simulink model "Power_Factor_Correction_using_CAPACITOR_BANK"  (R2022b)
settings: Solver=VariableStepAuto  StartTime=0.0  StopTime=0.2  RelTol=1e-3
undefined symbols (not defined in the file): D1, Delta
libraries: spsThreePhaseParallelRLCLoadLib x7, spsThreePhaseBreakerLib x6, spsPower3phInstantaneousLib x1, spsThreePhaseTransformerTwoWindingsLib x1, spsThreePhaseVIMeasurementLib x1, spsThreePhaseSourceLib x1, spspowerguiLib x1
settings Model: Creator=shubham  LastModifiedBy=shubham

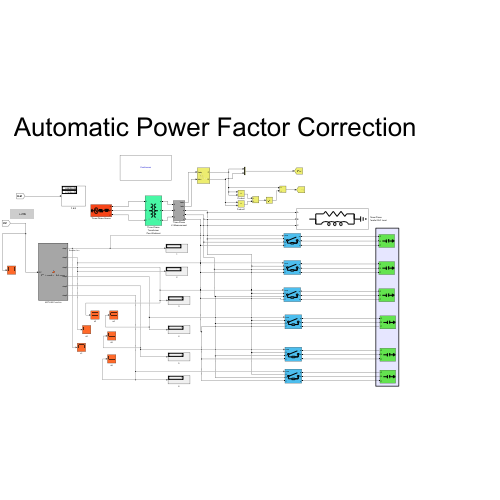
[thumbnail: Simulink's stored preview of the top-level diagram]
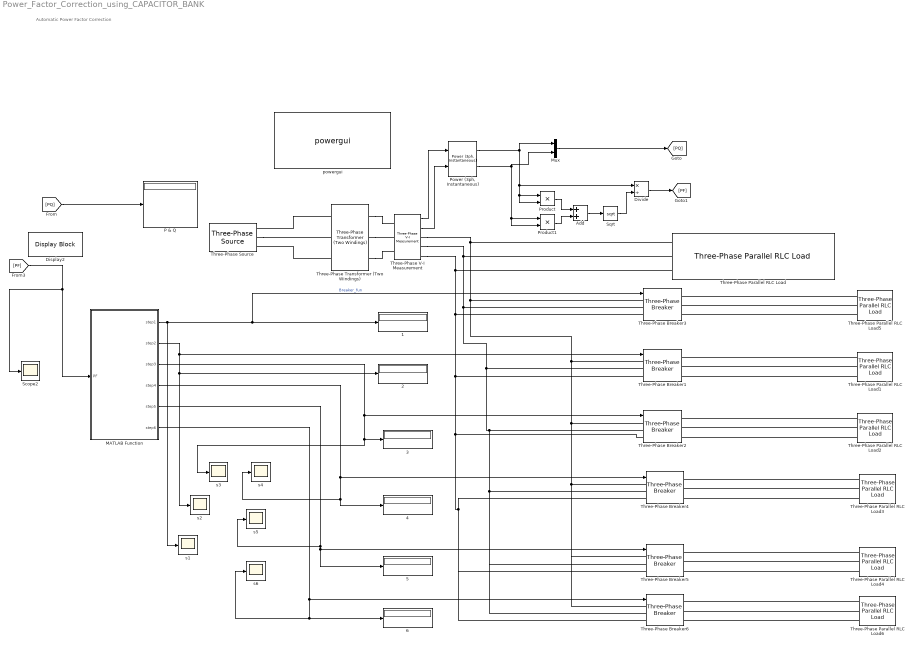
== system Power_Factor_Correction_using_CAPACITOR_BANK ==
  note: Automatic Power Factor Correction
  {1..6} (6 alike) : Display
      settings: Decimation=4
  Add : Sum
  Display2 : DisplayBlock  LabelPosition=Hide  Transparency=1  Layout=Fill available space
  Divide : Product  Inputs=*/
  MATLAB Function : MATLAB Function  TreatAsAtomicUnit=on
  Mux : Mux  Inputs=2
  P & Q : Display
      settings: Format=short_e  Decimation=4
  "Power (3ph, Instantaneous)" : spsPower3phInstantaneousLib/Power (3ph, Instantaneous)
  Product : Product
  Product1 : Product
  Scope2 : Scope
  Sqrt : Sqrt
  Three-Phase Parallel RLC Load : spsThreePhaseParallelRLCLoadLib/Three-Phase Parallel RLC Load  LConnTagsString=A|B|C  Configuration=Y (grounded)  NominalVoltage=6600  Vabc=[1e3 1e3 1e3]  Vabcp=[1e3 1e3 1e3]  NominalFrequency=50  UnbalancedPower=off  ActivePower=5000000  InductivePower=5845000  CapacitivePower=0  Pabc=[10e3 9e3 11e3]  QLabc=[100 90 110]  QCabc=[100 90 110]  Pabcp=[10e3 9e3 11e3]  QLabcp=[100 90 110]  QCabcp=[100 90 110]  Measurements=None  LoadType=constant Z
  Three-Phase Parallel RLC Load{1..6} (6 alike) : spsThreePhaseParallelRLCLoadLib/Three-Phase Parallel RLC Load  LConnTagsString=A|B|C  Configuration=Y (grounded)  NominalVoltage=6600  Vabc=[1e3 1e3 1e3]  Vabcp=[1e3 1e3 1e3]  NominalFrequency=50  UnbalancedPower=off  ActivePower=0  InductivePower=0  CapacitivePower=650000  Pabc=[10e3 9e3 11e3]  QLabc=[100 90 110]  QCabc=[100 90 110]  Pabcp=[10e3 9e3 11e3]  QLabcp=[100 90 110]  QCabcp=[100 90 110]  Measurements=None  LoadType=constant Z
  Three-Phase Transformer (Two Windings) : spsThreePhaseTransformerTwoWindingsLib/Three-Phase Transformer (Two Windings)  Winding1Connection=Delta (D1)  Winding2Connection=Yg  CoreType=Three single-phase transformers  SetSaturation=off  Hysteresis=off  DataFile='hysteresis'  SetInitialFlux=off  Measurements=None  UNITS=pu  NominalPower=[ 5e6 , 50 ]  Winding1=[ 33e3 , 0.002 , 0.08 ]  Winding2=[ 6.6e3 , 0.002 , 0.08 ]  Rm=500  Lm=500  L0=0.5  Saturation=[ 0,0 ; 0.0024,1.2 ; 1.0,1.52 ]  InitialFluxes=[ 0.8 , -0.8 , 0.7 ]  BreakLoop=off  DiscreteSolver=Trapezoidal iterative  DataType=off  TransfoNumber=1
  Three-Phase V-I Measurement : spsThreePhaseVIMeasurementLib/Three-Phase V-I Measurement  VoltageMeasurement=phase-to-ground  SetLabelV=off  LabelV=Vabc  Vpu=off  VpuLL=off  CurrentMeasurement=yes  SetLabelI=off  LabelI=Iabc  Ipu=off  Pbase=100e6  Vbase=500e3  OutputType=Complex  PhasorSimulation=off  PSBequivalent=0
  Three-Phase Breaker{1..6} (6 alike) : spsThreePhaseBreakerLib/Three-Phase Breaker  InitialState=open  SwitchA=on  SwitchB=on  SwitchC=on  SwitchTimes="[1/60  5/60]"  External=on  BreakerResistance=0.01  SnubberResistance=1e6  SnubberCapacitance=inf  Measurements=None
  Three-Phase Source : spsThreePhaseSourceLib/Three-Phase Source  InternalConnection=Yg  VoltagePhases=off  Voltage=33000  PhaseAngle=0  Voltage_phases=[25e3 25e3 25e3]/sqrt(3)  PhaseAngles_phases=[0 -120 +120]  Frequency=50  NonIdealSource=on  SpecifyImpedance=on  Resistance=0.8929  Inductance=16.58e-3  ShortCircuitLevel=100e6  BaseVoltage=25e3  XRratio=7  BusType=swing  Pref=10e3  Qref=0  Prefabc=[10e3, 10e3, 10e3]  Qrefabc=[0, 0, 0]  Qmin=-inf  Qmax=inf
  powergui : spspowerguiLib/powergui  Priority=1  SimulationMode=Continuous  SampleTime=50e-6  frequency=60  Iterations=50  frequencyindice=50  Pbase=100e6  ErrMax=1e-4  UnitsV=kV  UnitsW=MW  buscounter=0  FunctionMessages=off  echomessages=off  EnableUseOfTLC=off  CurrentSourceSwitches=off  DisableSnubberDevices=off  DisableRonSwitches=off  DisableVfSwitches=off  DisplayEquations=off  AutomaticDiscreteSolvers=off  SolverType=Tustin/Backward Euler (TBE)  Interpol=off  ExternalGateDelay=off  methode=off  Ts=100  x0status=blocks  SPID=on  SwTol=0  HookPort=off  NonlinearTolerance=1e-4  nMaxIteration=100  ContinueOnMaxIteration=off  RestoreLinks=warning  ResistiveCurrentMeasurement=off  Frange=[0:2:500]  Ylog=off  Xlog=on  ShowGrid=off  save=off  variable=ZData  structure=0  ZoomFFT=off  StartTime=0.0  cycles=1  DisplayStyle=1  fundamental=60  FreqAxis=off  MaxFrequency=1000  frequencyindicesteady=1  RmsSteady=1  display=off
  s{1..6} (6 alike) : Scope
  wires:
  "Power (3ph, Instantaneous)"/1 -> Mux/1, Product/2, Product/1, Divide/1
  Mux/1 -> [PQ]
  Sqrt/1 -> Divide/2
  Product1/1 -> Add/2
  Add/1 -> Sqrt/1
  Product/1 -> Add/1
  Three-Phase V-I Measurement/1 -> "Power (3ph, Instantaneous)"/1
  Three-Phase V-I Measurement/2 -> "Power (3ph, Instantaneous)"/2
  "Power (3ph, Instantaneous)"/2 -> Mux/2, Product1/2, Product1/1
  Divide/1 -> [PF]
  [PF] -> MATLAB Function/1(PF), Scope2/1
  MATLAB Function/1(step1) -> 1/1, Three-Phase Breaker3/1, s1/1  "Breaker_fun"
  [PQ] -> P & Q/1
  MATLAB Function/2(step2) -> s2/1, 2/1, Three-Phase Breaker1/1
  MATLAB Function/3(step3) -> s3/1, 3/1, Three-Phase Breaker2/1
  MATLAB Function/5(step5) -> 5/1, Three-Phase Breaker5/1, s5/1
  MATLAB Function/4(step4) -> 4/1, s4/1, Three-Phase Breaker4/1
  MATLAB Function/6(step6) -> s6/1, 6/1, Three-Phase Breaker6/1
  connections:
  Three-Phase Breaker4/LConn3 -- Three-Phase Breaker6/LConn3 -- Three-Phase Breaker5/LConn3 -- Three-Phase V-I Measurement/RConn3 -- Three-Phase Parallel RLC Load/LConn3 -- Three-Phase Breaker3/LConn3 -- Three-Phase Breaker1/LConn3 -- Three-Phase Breaker2/LConn3
  Three-Phase Breaker4/LConn2 -- Three-Phase Breaker6/LConn2 -- Three-Phase Breaker5/LConn2 -- Three-Phase V-I Measurement/RConn2 -- Three-Phase Parallel RLC Load/LConn2 -- Three-Phase Breaker3/LConn2 -- Three-Phase Breaker1/LConn2 -- Three-Phase Breaker2/LConn2
  Three-Phase Breaker4/LConn1 -- Three-Phase Breaker6/LConn1 -- Three-Phase Breaker5/LConn1 -- Three-Phase V-I Measurement/RConn1 -- Three-Phase Parallel RLC Load/LConn1 -- Three-Phase Breaker3/LConn1 -- Three-Phase Breaker1/LConn1 -- Three-Phase Breaker2/LConn1
  Three-Phase Transformer (Two Windings)/LConn3 -- Three-Phase Source/RConn3
  Three-Phase Transformer (Two Windings)/RConn2 -- Three-Phase V-I Measurement/LConn2
  Three-Phase Source/RConn2 -- Three-Phase Transformer (Two Windings)/LConn2
  Three-Phase Transformer (Two Windings)/LConn1 -- Three-Phase Source/RConn1
  Three-Phase Transformer (Two Windings)/RConn3 -- Three-Phase V-I Measurement/LConn3
  Three-Phase Transformer (Two Windings)/RConn1 -- Three-Phase V-I Measurement/LConn1
  Three-Phase Parallel RLC Load5/LConn2 -- Three-Phase Breaker3/RConn2
  Three-Phase Parallel RLC Load5/LConn1 -- Three-Phase Breaker3/RConn1
  Three-Phase Parallel RLC Load5/LConn3 -- Three-Phase Breaker3/RConn3
  Three-Phase Parallel RLC Load1/LConn1 -- Three-Phase Breaker1/RConn1
  Three-Phase Parallel RLC Load1/LConn2 -- Three-Phase Breaker1/RConn2
  Three-Phase Parallel RLC Load1/LConn3 -- Three-Phase Breaker1/RConn3
  Three-Phase Parallel RLC Load2/LConn2 -- Three-Phase Breaker2/RConn2
  Three-Phase Parallel RLC Load2/LConn1 -- Three-Phase Breaker2/RConn1
  Three-Phase Parallel RLC Load2/LConn3 -- Three-Phase Breaker2/RConn3
  Three-Phase Parallel RLC Load4/LConn1 -- Three-Phase Breaker5/RConn1
  Three-Phase Parallel RLC Load3/LConn1 -- Three-Phase Breaker4/RConn1
  Three-Phase Parallel RLC Load3/LConn3 -- Three-Phase Breaker4/RConn3
  Three-Phase Parallel RLC Load4/LConn2 -- Three-Phase Breaker5/RConn2
  Three-Phase Parallel RLC Load4/LConn3 -- Three-Phase Breaker5/RConn3
  Three-Phase Parallel RLC Load3/LConn2 -- Three-Phase Breaker4/RConn2
  Three-Phase Parallel RLC Load6/LConn2 -- Three-Phase Breaker6/RConn2
  Three-Phase Parallel RLC Load6/LConn1 -- Three-Phase Breaker6/RConn1
  Three-Phase Parallel RLC Load6/LConn3 -- Three-Phase Breaker6/RConn3

== matlab function Power_Factor_Correction_using_CAPACITOR_BANK/MATLAB Function ==
  data: PF input; step1 output; step2 output; step3 output; step4 output; step5 output; step6 output
function [step1, step2, step3, step4, step5, step6] = PF_Capacitor_Switching(PF)
    % Target power factor
    target_PF = 0.95;
    
    % Initialize all steps to OFF (0)
    step1 = 0;
    step2 = 0;
    step3 = 0;
    step4 = 0;
    step5 = 0;
    step6 = 0;
    
    % Turn ON capacitors based on PF thresholds
    if PF < target_PF
        % Step 1: Always ON if PF < 0.95
        step1 = 1;
        
        % Step 2: ON if PF < 0.90
        if PF < 0.90
            step2 = 1;
        end
        
        % Step 3: ON if PF < 0.85
        if PF < 0.88
            step3 = 1;
        end
        
        % Step 4: ON if PF < 0.80
        if PF < 0.85
            step4 = 1;
        end
        
        % Step 5: ON if PF < 0.75
        if PF < 0.83
            step5 = 1;
        end
        
        % Step 6: ON if PF < 0.70
        if PF < 0.80
            step6 = 1;
        end
    end
end
